simulink model "apilot1"  (Simulink 3.00)
settings: Solver=ode15s  SolverMode=SingleTasking  StartTime=0.0  StopTime=100  MaxStep=2  RelTol=1e-06  AbsTol=1e-04
undefined symbols (not defined in the file): sfunyst
libraries: aplib x8, fbuttons x3, fdclib10 x1
settings Model: SaveTime=off  SaveOutput=off  RTWTemplateMakefile=grt_vc.tmf  LastModifiedBy=Dutchroll

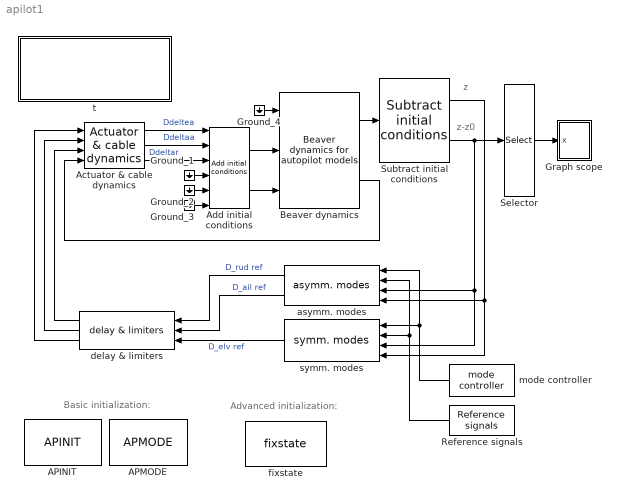
== system apilot1 ==
  note: z-z0
  note: z
  note: Basic initialization:
  note: Advanced initialization:
  APINIT : fbuttons/APINIT
  APMODE : fbuttons/APMODE
  Actuator & cable dynamics : aplib/Actuator & cable dynamics
  Add initial conditions : aplib/Add initial conditions
  Beaver dynamics : fdclib10/Beaver dynamics for autopilot models
  Graph scope : Subsystem  mask(Storage scope.){npts=100, color='g-'}
      mask prompts: npts "Initial Time Range:"; color "Initial y-min:"
      mask help:
      | Storage scope using MATLAB graph window.
      | Enter plotting ranges and line type.
      mask init:
      | close all; ax = [0, @1, @2, @3];
      mask Help: Uses MATLAB's graph window.\nUse only one block per system.\nLine type must be in quotes.\nSee the M-file sfunyst.m.
      mask Display: plot(0,0,100,100,[83,76,63,52,42,38,28,16,11,84,11,11,11,90,90,11],[75,58,47,54,72,80,84,74,65,65,65,90,40,40,90,90])
  Ground_{1..4} (4 alike) : Ground
  Reference signals : aplib/Reference signals  Orientation=left
  Selector : Selector  Elements=8  InputPortWidth=13
  Subtract initial conditions : aplib/Subtract initial conditions
  asymm. modes : aplib/asymm. modes  Orientation=left
  delay & limiters : aplib/delay & limiters  Orientation=left
  fixstate : fbuttons/fixstate
  mode controller : aplib/mode controller  Orientation=left
  symm. modes : aplib/symm. modes  Orientation=left
  t : Subsystem
      settings: OpenFcn=browse apilot
      mask Display: disp('Apilot1 (no radio-navigation,\nwind, turbulence, and\nsensor models)\nMarc Rauw, April 2004')
  wires:
  Add initial conditions/2 -> Beaver dynamics/3
  Add initial conditions/1 -> Beaver dynamics/2
  Beaver dynamics/1 -> Subtract initial conditions/1
  delay & limiters/2 -> Actuator & cable dynamics/2
  delay & limiters/3 -> Actuator & cable dynamics/1
  symm. modes/1 -> delay & limiters/3  "D_elv ref"
  Subtract initial conditions/1 -> symm. modes/4, asymm. modes/4
  Reference signals/1 -> asymm. modes/2, symm. modes/2
  Subtract initial conditions/2 -> symm. modes/3, asymm. modes/3, Selector/1
  asymm. modes/1 -> delay & limiters/1  "D_rud ref"
  asymm. modes/2 -> delay & limiters/2  "D_ail ref"
  Beaver dynamics/2 -> Actuator & cable dynamics/4
  mode controller/1 -> asymm. modes/1, symm. modes/1
  Ground_1/1 -> Add initial conditions/4
  Ground_2/1 -> Add initial conditions/5
  Ground_3/1 -> Add initial conditions/6
  Actuator & cable dynamics/1 -> Add initial conditions/1  "Ddeltea"
  Actuator & cable dynamics/2 -> Add initial conditions/2  "Ddeltaa"
  Actuator & cable dynamics/3 -> Add initial conditions/3  "Ddeltar"
  delay & limiters/1 -> Actuator & cable dynamics/3
  Ground_4/1 -> Beaver dynamics/1
  Selector/1 -> Graph scope/1(x)

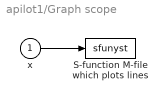
== system apilot1/Graph scope ==
  x : Inport  Port=1  PortWidth=-1  SampleTime=-1  DataType=auto
      settings: SignalType=auto
  "S-function M-file which plots lines " : S-Function  LoadFcn=sfunyst([],[],[],'LoadBlock')  FunctionName=sfunyst  Parameters=ax, color, npts  PortCounts=[]  SFunctionModules=''
      settings: CopyFcn=sfunyst([],[],[],'CopyBlock')  DeleteFcn=sfunyst([],[],[],'DeleteBlock')
  wires:
  x/1 -> "S-function M-file which plots lines "/1

== system apilot1/t ==
